simulink model "top_model"  (R2017a)
settings: Solver=VariableStepAuto  StartTime=0.0  StopTime=inf  RelTol=1e-3  EnableMultiTasking=on
undefined symbols (not defined in the file): acceptanceR, Aref, Bref, craftSpeedCurvatureLookup, kobuki, lookAheadDistance, obstacleList, pathCurvature, Psi0, setState, target, x0, y0
libraries: simulink x1
settings Model: Creator=The MathWorks, Inc.  LastModifiedBy=Max
settings DataIOCC: LimitDataPoints=on
settings OptimizationCC: LifeSpan=inf
settings DebuggingCC: AllowSymbolicDim=off  SFUnexpectedBacktrackingDiag=warning  SFNoUnconditionalDefaultTransitionDiag=warning  SFExecutionAtInitializationDiag=none
settings ModelReferenceCC: EnableParallelModelReferenceBuilds=on  PropagateSignalLabelsOutOfModel=off
settings GRTTargetCC: TargetLangStandard=C89/C90 (ANSI)
settings ConfigComp: CovMetricSettings=dw  CovHtmlReporting=on  CovSaveCumulativeToWorkspaceVar=on  CovSaveSingleToWorkspaceVar=on  CovExternalEMLEnable=off

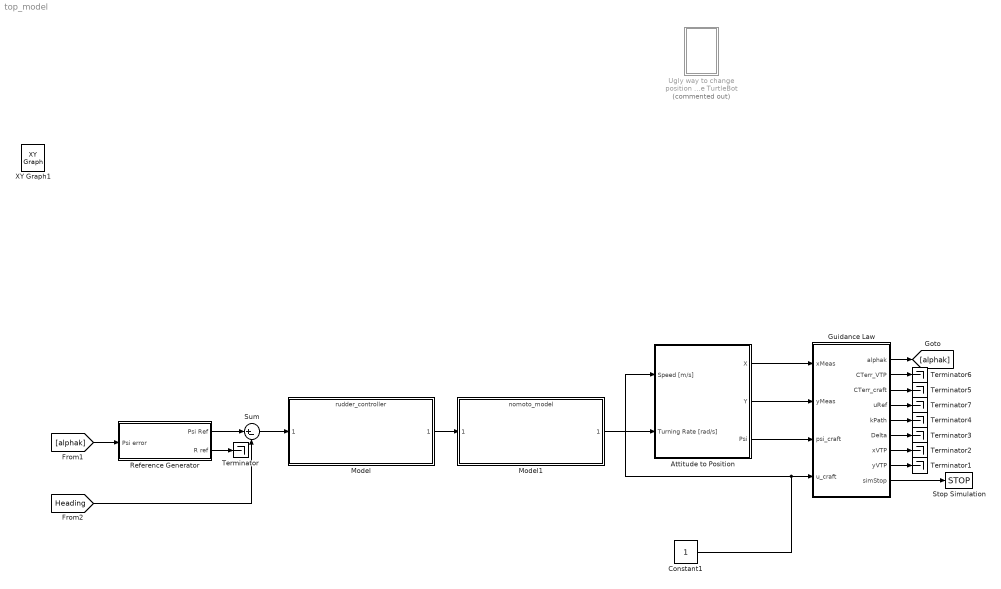
== system top_model ==
  Attitude to Position : Subsystem
  Constant1 : Constant
  Guidance Law : MATLAB Function  TreatAsAtomicUnit=on
  Model : ModelReference  ModelNameDialog=rudder_controller  SimulationMode=Normal  ModelReferenceVersion=1.1
  Model1 : ModelReference  ModelNameDialog=nomoto_model  SimulationMode=Normal  ModelReferenceVersion=1.8
  Reference Generator : Subsystem
  Stop Simulation : Stop
  Sum : Sum  Inputs=|+-
  Terminator{,1..7} (8 alike) : Terminator
  Ugly way to change position of the TurtleBot : Subsystem  Commented=on
  XY Graph1 : simulink/Sinks/XY Graph  IOType=viewer  xmin=0  xmax=200  ymin=0  ymax=200  st=-1
  wires:
  Model1/1 -> Attitude to Position/2(Turning Rate [rad/s])
  Guidance Law/9(simStop) -> Stop Simulation/1
  Attitude to Position/1(X) -> Guidance Law/1(xMeas)
  Attitude to Position/2(Y) -> Guidance Law/2(yMeas)
  [alphak] -> Reference Generator/1(Psi error)
  Guidance Law/1(alphak) -> [alphak]
  [Heading] -> Sum/2
  Reference Generator/1(Psi Ref) -> Sum/1
  Sum/1 -> Model/1
  Reference Generator/2(R ref) -> Terminator/1
  Model/1 -> Model1/1
  Guidance Law/8(yVTP) -> Terminator1/1
  Guidance Law/7(xVTP) -> Terminator2/1
  Guidance Law/6(Delta) -> Terminator3/1
  Guidance Law/5(kPath) -> Terminator4/1
  Guidance Law/3(CTerr_craft) -> Terminator5/1
  Guidance Law/2(CTerr_VTP) -> Terminator6/1
  Attitude to Position/3(Psi) -> Guidance Law/3(psi_craft)
  Constant1/1 -> Attitude to Position/1(Speed [m/s]), Guidance Law/4(u_craft)
  Guidance Law/4(uRef) -> Terminator7/1

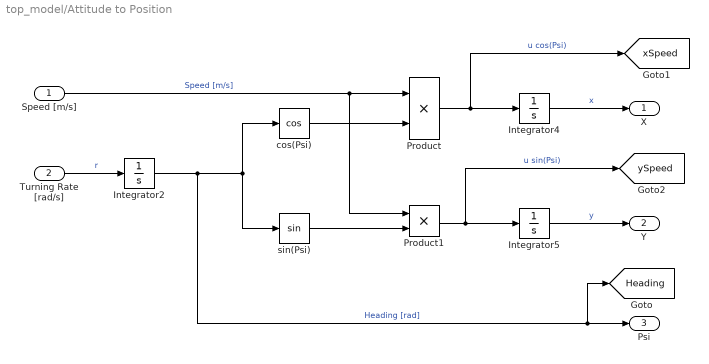
== system top_model/Attitude to Position ==
  Speed [m/s] : Inport
  Turning Rate [rad/s] : Inport  Port=2
  Integrator2 : Integrator  Priority=3  InitialCondition=Psi0  ContinuousStateAttributes='craft_Psi'
  Integrator4 : Integrator  Priority=1  InitialCondition=x0  ContinuousStateAttributes='craft_x'
  Integrator5 : Integrator  Priority=2  InitialCondition=y0  ContinuousStateAttributes='craft_y'
  Product : Product
  Product1 : Product
  cos(Psi) : Trigonometry  Operator=cos
  sin(Psi) : Trigonometry
  X : Outport
  Y : Outport  Port=2
  Psi : Outport  Port=3
  tag scope: Heading=global, xSpeed=global, ySpeed=global
  wires:
  Product1/1 -> [ySpeed], Integrator5/1  "u sin(Psi)"
  Product/1 -> [xSpeed], Integrator4/1  "u cos(Psi)"
  Speed [m/s]/1 -> Product1/1, Product/1  "Speed [m/s]"
  Turning Rate [rad/s]/1 -> Integrator2/1  "r"
  Integrator4/1 -> X/1  "x"
  sin(Psi)/1 -> Product1/2
  Integrator5/1 -> Y/1  "y"
  cos(Psi)/1 -> Product/2
  Integrator2/1 -> [Heading], Psi/1, cos(Psi)/1, sin(Psi)/1  "Heading [rad]"

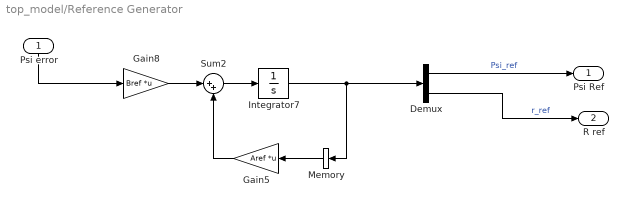
== system top_model/Reference Generator ==
  Psi error : Inport
  Demux : Demux  Outputs=2
  Gain5 : Gain  Gain=Aref  Multiplication=Matrix(K*u) (u vector)
  Gain8 : Gain  Gain=Bref  Multiplication=Matrix(K*u) (u vector)
  Integrator7 : Integrator  Priority=99  InitialCondition=[Psi0;0]  ContinuousStateAttributes='craft_r'
  Memory : Memory  InheritSampleTime=on
  Sum2 : Sum  Inputs=|++
  Psi Ref : Outport
  R ref : Outport  Port=2
  wires:
  Demux/1 -> Psi Ref/1  "Psi_ref"
  Gain8/1 -> Sum2/1
  Integrator7/1 -> Demux/1, Memory/1
  Gain5/1 -> Sum2/2
  Sum2/1 -> Integrator7/1
  Demux/2 -> R ref/1  "r_ref"
  Psi error/1 -> Gain8/1
  Memory/1 -> Gain5/1

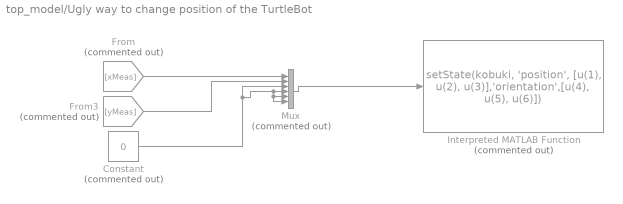
== system top_model/Ugly way to change position of the TurtleBot ==
  Constant : Constant  Commented=on  Value=0
  From : From  Commented=on  GotoTag=xMeas
  From3 : From  Commented=on  GotoTag=yMeas
  Interpreted MATLAB Function : MATLABFcn  Commented=on  MATLABFcn=setState(kobuki, 'position', [u(1), u(2), u(3)],'orientation',[u(4), u(5), u(6)])  OutputDimensions=0
  Mux : Mux  Commented=on  Inputs=6
  wires:
  Mux/1 -> Interpreted MATLAB Function/1
  From/1 -> Mux/1
  From3/1 -> Mux/2
  Constant/1 -> Mux/6, Mux/5, Mux/4, Mux/3

== matlab function top_model/Guidance Law ==
  data: alphak output double; xMeas input; yMeas input; obstacleList parameter; target parameter; CTerr_VTP output; lookAheadDistance parameter; pathCurvature parameter; acceptanceR parameter; craftSpeedCurvatureLookup parameter; psi_craft input; u_craft input; CTerr_craft output; uRef output; kPath output; Delta output; xVTP output; yVTP output; simStop output
function [alphak,CTerr_VTP, CTerr_craft, uRef, kPath, Delta, xVTP, yVTP, simStop] = fcn(xMeas, yMeas, obstacleList, target, lookAheadDistance, pathCurvature, acceptanceR, craftSpeedCurvatureLookup, psi_craft, u_craft)
coder.extrinsic('tic');
coder.extrinsic('toc');
coder.extrinsic('evalin');
coder.extrinsic('disp');
coder.extrinsic('get_param');
coder.extrinsic('strcat');
coder.extrinsic('num2str');
coder.extrinsic('assignin');

%% 17/02/15 - attempt to implement variable lookahead reference from curvature
% attempt to add variable speed control from curvature

persistent trajectory trajX trajY trigger calculated tanCurve prevAlphaK turnCounter lookAheadDistanceP baseLookAheadDistance iTarget

% deal with missing data
if isempty(trigger)
    trigger = obstacleList(:,3);
end

%if isempty(baseLookAheadDistance)
    baseLookAheadDistance = 25;
%end;
if isempty(iTarget)
    iTarget = 1;
end

if (iTarget > length(target))
    simStop = 1;
    iTarget = length(target);
end
if isempty(lookAheadDistanceP)
    lookAheadDistanceP = 0;
end

if isempty(calculated)
    calculated = obstacleList(:,3);
end

if isempty(trajectory)
    tx = target(iTarget,1);
    ty = target(iTarget,2);
    [trajX,trajY] = getTrajectory(xMeas, yMeas, tx,ty, obstacleList);
    trajectory = [trajX, trajY];
end

% if isempty(pathCurvature)
%     pathCurvature = CurvatureEstimation(trajectory); % NOT SUPPORTED IN
%     CODE GENERATION, USE ALTERNATIVE FUNCTION TO GET CURVATURE, FOR NOW
%     IT IS JUST PRECOMPUTED BEFORE RUNNING
% end

if isempty(tanCurve)
        tanCurve = atan2(trajY,trajX);
end

if isempty(prevAlphaK)
    prevAlphaK = 0;
end

if isempty(turnCounter)
    turnCounter = 0;
end


% Check cross track error between craft and path
dx = trajX - xMeas;
dy = trajY - yMeas;
[CTerr_craft, ind_craft] = min(hypot(dx, dy));


% Create Virtual Target ahead (first case to check the curvature)
VTP = [xMeas+lookAheadDistance*cos(psi_craft), yMeas+lookAheadDistance*sin(psi_craft)];
xVTP = VTP(1);
yVTP = VTP(2);



% Check cross track error between VTP and path
dx = trajX - VTP(1);
dy = trajY - VTP(2);
[~, ind_VTP] = min(hypot(dx, dy));

% Redraw particle according to curvature
lookAheadDistance = baseLookAheadDistance - 650*max(pathCurvature(ind_VTP),pathCurvature(ind_craft));
if (lookAheadDistance<5)
    lookAheadDistance = 5;
end
if isnan(lookAheadDistance)
    lookAheadDistance = baseLookAheadDistance;
end
Delta = lookAheadDistance;
VTP = [xMeas+Delta*cos(psi_craft),yMeas+Delta*sin(psi_craft)];
xVTP = VTP(1);
yVTP = VTP(2);
% Check cross track error between new VTP and path
dx = trajX - VTP(1);
dy = trajY - VTP(2);
[CTerr_VTP, ind_VTP] = min(hypot(dx, dy));
VTP_projection = [trajX(ind_VTP),trajY(ind_VTP)];

% angleTangent = tanCurve(ind_VTP);
% pLOS = [VTP_projection(1)+lookAheadDistanceP*cos(angleTangent),VTP_projection(2)+lookAheadDistanceP*sin(angleTangent)];

% Reference angle is the vector that points from the craft to the
% projection of the VTP on the track
alphak = atan2(VTP_projection(2)-yMeas,VTP_projection(1)-xMeas);



% Calculate cross-track errors
% Find out if the craft is on one side or the other
angle1 = atan2(trajY(ind_craft)-trajY(1),trajX(ind_craft)-trajX(1));
angle2 = atan2(yMeas-trajY(1),xMeas-trajX(1));
if (angle2<angle1) % Craft inside the curve
    CTerr_craft = -CTerr_craft;
end

% Find out if the VPT is on one side or the other
angle1 = atan2(trajY(ind_VTP)-trajY(1),trajX(ind_VTP)-trajX(1));
angle2 = atan2(VTP(2)-trajY(1),VTP(1)-trajX(1));
if (angle2<angle1) % Craft inside the curve
   CTerr_VTP = -CTerr_VTP;
end

%% Alternative (traditional LOS) the particle is on the tangent of the path

% craftProjection = [trajX(ind_craft),trajY(ind_craft)];
% angleTangent = tanCurve(ind_craft);
% pLOS = [craftProjection(1)+lookAheadDistance*cos(angleTangent),craftProjection(2)+lookAheadDistance*sin(angleTangent)];

% alphak = atan2(pLOS(2)-yMeas,pLOS(1)-xMeas);
% alphak = alphak - turnCounter*2*pi;
%% Correct angle jumps (TODO: CHECK properly)

if ((abs(prevAlphaK-alphak)>pi)) % a tan discontinuity happened
    if (alphak>prevAlphaK)   
         alphak = alphak - 2*pi;
         turnCounter = turnCounter + 1;
    else
         alphak = alphak + 2*pi;
         turnCounter = turnCounter - 1;
    end
        
end
   
prevAlphaK = alphak;

% Curvature -> speed reference, it takes the maximum curvature between the
% craft and the particle (conservative)
maxCurvature = max(pathCurvature(ind_craft),pathCurvature(ind_VTP)); 
uRef = interp1(craftSpeedCurvatureLookup(:,2),craftSpeedCurvatureLookup(:,1),maxCurvature);
kPath = pathCurvature(ind_craft);

xTarget = target(iTarget, 1);
yTarget = target(iTarget, 2);
%% Vtp to target distance
distance = ((xTarget - xMeas)^2 + (yTarget - yMeas)^2)^0.5;
if (distance < 5)
    iTarget = min(iTarget +1,length(target)+1) ; 
    trajectory = [];
end

simStop = 0;
if (iTarget > length(target))
    simStop = 1;
end
end
